simulink model "mobile_robot"  (R2022a)
settings: Solver=VariableStepAuto  StartTime=0.0  StopTime=10.0  RelTol=1e-3
values from neighbouring files (symbols this model uses):
  b = .1    (= 0.1)    [robotScript.m]
settings Model: Creator=natha  LastModifiedBy=natha

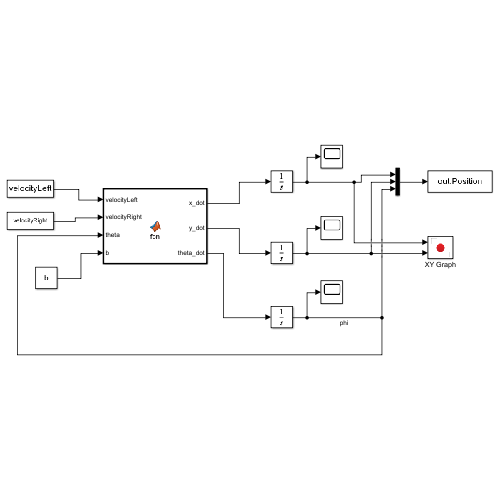
[thumbnail: Simulink's stored preview of the top-level diagram]
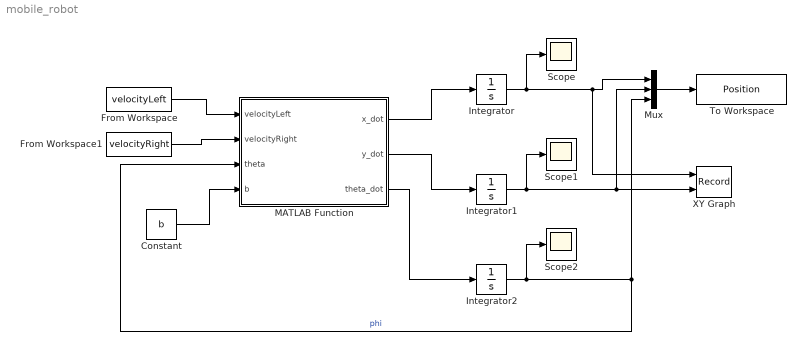
== system mobile_robot ==
  Constant : Constant  Value=b
  From Workspace : FromWorkspace  VariableName=velocityLeft
  From Workspace1 : FromWorkspace  VariableName=velocityRight
  Integrator : Integrator
  Integrator1 : Integrator
  Integrator2 : Integrator
  MATLAB Function : MATLAB Function  TreatAsAtomicUnit=on
  Mux : Mux  Inputs=3
  Scope : Scope
  Scope1 : Scope
  Scope2 : Scope
  To Workspace : ToWorkspace  VariableName=Position  SaveFormat=Timeseries  SampleTime=-1
  XY Graph : Record  FileSettingsInternal="{\"entries\":[{\"content\":{\"excelSettings\":{\"content\":{},\"type\":\"Streamout.ExcelSettings\"}},\"type\":\"Streamout.FileSettingStorage\",\"uuid\":\"92d81772-3c03-4705-be13-2119302ef6d8\"}],\"packageUris\":[\"http://schema.mathworks.com/mf0/streamout_blocks/R2020a\"],\"version\":\"1.0\"}"  Layout=[1 1]  SignalsInternal="{\"entries\":[{\"content\":{\"signals\":[{\"content\":{\"blockPath\":[\"mobile_robot/XY Graph\"],\"channel\":[],\"dimensions\":[1],\"domain\":\"mobile_robot/XY Graph\",\"lineColor\":\"#a2142f\",\"plots\":[1],\"port\":1,\"sid\":[\"\"],\"signalID\":49,\"signalName\":\"Integrator\"},\"type\":\"RecordBlkView.Signal\",\"uuid\":\"46e06312-3278-4392-86fe-22bbb21a408e\"},{\"content\":{\"blockPath\":[\"mobile_robot/XY Graph\"],\"channel\":[],\"dimensions\":[1],\"domain\":\"mobile_robot/XY Graph\",\"lineColor\":\"#139fff\",\"plots\":[1],\"port\":2,\"sid\":[\"\"],\"signalID\":53,\"signalName\":\"Integrator1\"},\"type\":\"RecordBlkView.Signal\",\"uuid\":\"0a380d3e-e626-4d9f-9f65-d38b0ff10dd6\"}]},\"type\":\"RecordBlkView.InputSignals\",\"uuid\":\"f47ccacc-b6e8-4195-90f7-c57acd015902\"}],\"packageUris\":[\"http://schema.mathworks.com/mf0/streamout_blocks/R2020a\"],\"version\":\"1.0\"}"  VisualizationBindings="{\"xyplotplugin\":{\"info\":[{\"series\":[{\"bindingParametersList\":[{\"parameter\":\"X-Axis\",\"signalID\":49,\"signalName\":\"Integrator\"},{\"parameter\":\"Y-Axis\",\"signalID\":53,\"signalName\":\"Integrator1\"}],\"seriesID\":2746}],\"subplotID\":1}]}}"  CompatibilityTag=XY
  wires:
  MATLAB Function/1(x_dot) -> Integrator/1
  Integrator/1 -> Scope/1, Mux/1, XY Graph/1
  Constant/1 -> MATLAB Function/4(b)
  MATLAB Function/2(y_dot) -> Integrator1/1
  Integrator1/1 -> XY Graph/2, Mux/2, Scope1/1
  MATLAB Function/3(theta_dot) -> Integrator2/1
  Integrator2/1 -> Mux/3, MATLAB Function/3(theta), Scope2/1  "phi"
  Mux/1 -> To Workspace/1
  From Workspace1/1 -> MATLAB Function/2(velocityRight)
  From Workspace/1 -> MATLAB Function/1(velocityLeft)

== matlab function mobile_robot/MATLAB Function ==
  data: velocityLeft input; velocityRight input; theta input; x_dot output; b input; y_dot output; theta_dot output
function [x_dot, y_dot, theta_dot] = fcn(velocityLeft, velocityRight, theta, b)

x_dot = cos(theta)*(velocityLeft + velocityRight)/2;
y_dot = sin(theta)*(velocityLeft + velocityRight)/2;
theta_dot = (velocityRight - velocityLeft)/b
